simulink model "ctrl_beta_nn"  (R2017a)
settings: Solver=FixedStepAuto  StartTime=0.0  StopTime=20  FixedStep=.001  RelTol=1e-3  EnableMultiTasking=on
settings Model: Creator=aaa  LastModifiedBy=aaa
settings OptimizationCC: LifeSpan=1
settings DebuggingCC: SFExecutionAtInitializationDiag=none

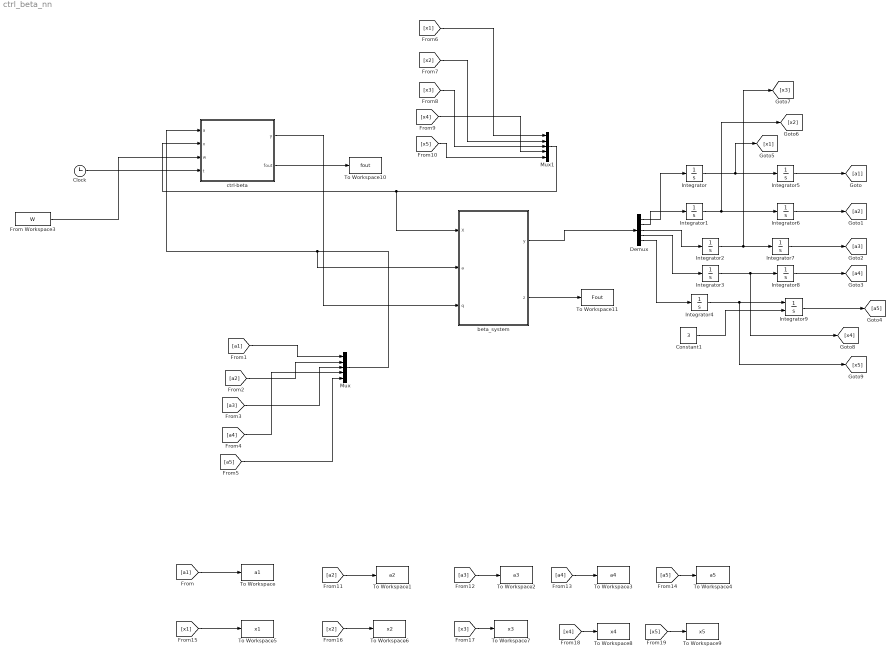
== system ctrl_beta_nn ==
  Clock : Clock
  Constant1 : Constant  Value=3
  Demux : Demux  Outputs=[1 1 1 1 1]
  From Workspace3 : FromWorkspace  VariableName=W  SampleTime=0
  Integrator : Integrator
  Integrator1 : Integrator
  Integrator2 : Integrator  InitialCondition=3.05
  Integrator3 : Integrator  InitialCondition=3
  Integrator4 : Integrator  InitialCondition=1
  Integrator5 : Integrator  InitialCondition=1
  Integrator6 : Integrator  InitialCondition=1
  Integrator7 : Integrator  InitialCondition=pi/6
  Integrator8 : Integrator  InitialCondition=pi/6*5
  Integrator9 : Integrator  InitialConditionSource=external
  Mux : Mux  Inputs=[1 1 1 1 1]
  Mux1 : Mux  Inputs=[1 1 1 1 1]
  To Workspace : ToWorkspace  VariableName=a1  SaveFormat=Timeseries  SampleTime=-1
  To Workspace1 : ToWorkspace  VariableName=a2  SaveFormat=Timeseries  SampleTime=-1
  To Workspace10 : ToWorkspace  VariableName=fout  SaveFormat=Timeseries  SampleTime=-1
  To Workspace11 : ToWorkspace  VariableName=Fout  SaveFormat=Timeseries  SampleTime=-1
  To Workspace2 : ToWorkspace  VariableName=a3  SaveFormat=Timeseries  SampleTime=-1
  To Workspace3 : ToWorkspace  VariableName=a4  SaveFormat=Timeseries  SampleTime=-1
  To Workspace4 : ToWorkspace  VariableName=a5  SaveFormat=Timeseries  SampleTime=-1
  To Workspace5 : ToWorkspace  VariableName=x1  SaveFormat=Timeseries  SampleTime=-1
  To Workspace6 : ToWorkspace  VariableName=x2  SaveFormat=Timeseries  SampleTime=-1
  To Workspace7 : ToWorkspace  VariableName=x3  SaveFormat=Timeseries  SampleTime=-1
  To Workspace8 : ToWorkspace  VariableName=x4  SaveFormat=Timeseries  SampleTime=-1
  To Workspace9 : ToWorkspace  VariableName=x5  SaveFormat=Timeseries  SampleTime=-1
  beta_system : MATLAB Function  TreatAsAtomicUnit=on
  ctrl-beta : MATLAB Function  TreatAsAtomicUnit=on
  wires:
  ctrl-beta/1(y) -> beta_system/3(q)
  Integrator8/1 -> [a4]
  [a3] -> To Workspace2/1
  Integrator6/1 -> [a2]
  From Workspace3/1 -> ctrl-beta/3(w)
  [a4] -> To Workspace3/1
  Integrator9/1 -> [a5]
  [x2] -> Mux1/2
  Integrator3/1 -> [x4], Integrator8/1
  Integrator/1 -> [x1], Integrator5/1
  [x4] -> Mux1/4
  Integrator7/1 -> [a3]
  Mux1/1 -> ctrl-beta/2(x), beta_system/1(X)
  Demux/1 -> Integrator/1
  [a4] -> Mux/4
  [a5] -> Mux/5
  Integrator4/1 -> [x5], Integrator9/1
  Demux/5 -> Integrator4/1
  [a5] -> To Workspace4/1
  [x3] -> To Workspace7/1
  [x4] -> To Workspace8/1
  [a2] -> Mux/2
  [x5] -> To Workspace9/1
  Integrator5/1 -> [a1]
  [a2] -> To Workspace1/1
  [x1] -> Mux1/1
  Demux/4 -> Integrator3/1
  [a3] -> Mux/3
  Demux/3 -> Integrator2/1
  Integrator1/1 -> [x2], Integrator6/1
  [x1] -> To Workspace5/1
  beta_system/1(y) -> Demux/1
  [x3] -> Mux1/3
  Integrator2/1 -> [x3], Integrator7/1
  [a1] -> Mux/1
  Constant1/1 -> Integrator9/2
  [x5] -> Mux1/5
  [a1] -> To Workspace/1
  Mux/1 -> ctrl-beta/1(a), beta_system/2(a)
  Demux/2 -> Integrator1/1
  [x2] -> To Workspace6/1
  ctrl-beta/2(fout) -> To Workspace10/1
  beta_system/2(z) -> To Workspace11/1
  Clock/1 -> ctrl-beta/4(t)

== matlab function ctrl_beta_nn/ctrl-beta ==
  data: a input; x input; y output; w input; fout output; t input
function [y,fout] = fcn(a,x,w,t)

a5=a(5);
x5=x(5);
X=zeros(8,1);
X(1:2)=a(1:2);X(3)=a(5); X(4:8)=x;

num=length(w)-1;
c=X*(1+((1:num)-(num+1)/2)*.05);
sig=sqrt(num+1)/.05;
p=NaN(num,1);
for i=1:num, p(i)=exp(-(X-c(:,i))'*(X-c(:,i))*(sig^2)); end
aaa=0;
fout=w'*[p;1];
y=-10*(x5-aaa)-10*(a5-aaa*t)+fout;

== matlab function ctrl_beta_nn/beta_system ==
  data: X input; y output; a input; q input; z output
function [y,z] = fcn(X,a,q)
% function y = fcn(X,a)
x1=X(1);%dL1
x2=X(2);%dL2
x3=X(3);%dth1
x4=X(4);%dth2
x5=X(5);%dbeta
%NO-Derivative variables as parameters
a1=a(1);a2=a(2);a3=a(3);a4=a(4);a5=a(5);
%other terms
E=1e4; A=1; m=100; w=0.0011; ello=500;
K=E*A/(m*w^2*ello);
th=a3-a4;
L3=(a1^2+a2^2+2*a1*a2*cos(th))^0.5;
e1=1*(a1>1)+0*(a1<=1);
e2=1*(a2>1)+0*(a2<=1);
e3=1*(L3>1)+0*(L3<=1);

%equation
M=[2 cos(th) 0 a2*sin(th) 0;
    cos(th) 2 -a1*sin(th) 0 0;
    0 -a1*sin(th) 2*a1^2 a1*a2*cos(th) 0;
    a2*sin(th) 0 a1*a2*cos(th) 2*a2^2 0;
    0 0 0 0 2*(a1^2*cos(a3)^2+a2^2*cos(a4)^2+a1*a2*cos(a3)*cos(a4))];
N=[2*sin(th)*cos(a5)*x2-2*a1*x3*(x3+2*cos(a5))-a2*cos(a5)*x4*(2*cos(a5)+x4)-(2*a1*cos(a3)+a2*cos(a4))*...
    (2*sin(a5)*sin(a3)+cos(a3)*x5)*x5+2*sin(th)*x2*x4;
    -2*sin(th)*cos(a5)*x1-2*a2*x4*(x4+2*cos(a5))-a1*cos(a5)*x3*(2*cos(a5)+x3)-(2*a2*cos(a4)+a1*cos(a3))*...
    (2*sin(a5)*sin(a4)+cos(a4)*x5)*x5-2*sin(th)*x1*x3;
    4*cos(a5)*a1*x1+2*cos(a5)^2*a1*x2+a1*a2*sin(th)*x4*(2*cos(a5)+x4)+(2*a1*cos(a3)+a2*cos(a4))*...
    (a1*sin(a3)*x5-2*a1*cos(a3)*sin(a5))*x5+4*a1*x1*x3+2*a1*cos(a5)*x2*x4;
    4*cos(a5)*a2*x2+2*cos(a5)^2*a2*x1-a1*a2*sin(th)*x3*(2*cos(a5)+x3)+(2*a2*cos(a4)+a1*cos(a3))*...
    (a2*sin(a4)*x5-2*a2*cos(a4)*sin(a5))*x5+4*a2*x2*x4+2*a2*cos(a5)*x1*x3;
    2*sin(a3)*sin(a5)*(2*a1*cos(a3)+a2*cos(a4))*x1+2*sin(a4)*sin(a5)*(2*a2*cos(a4)+a1*cos(a3))*x2+...
    2*a1*cos(a3)*sin(a5)*(2*a1*cos(a3)+a2*cos(a4))*x3+2*a2*cos(a4)*sin(a5)*(2*a2*cos(a4)+a1*cos(a3))*x4+...
    2*(2*a1*cos(a3)+a2*cos(a4))*cos(a3)*x5*x1+2*(2*a2*cos(a4)+a1*cos(a3))*cos(a4)*x5*x2-...
    2*(2*a1*cos(a3)+a2*cos(a4))*a1*sin(a3)*x3*x5-2*(2*a2*cos(a4)+a1*cos(a3))*a2*sin(a4)*x4*x5];
G=[-cos(a3)*(2*a1*cos(a3)+a2*cos(a4))*(1+2*cos(2*a5));
    -cos(a4)*(2*a2*cos(a4)+a1*cos(a3))*(1+2*cos(2*a5));
    a1*sin(a3)*(2*a1*cos(a3)+a2*cos(a4))*(1+2*cos(2*a5));
    a2*sin(a4)*(2*a2*cos(a4)+a1*cos(a3))*(1+2*cos(2*a5));
    4*(a1^2*cos(a3)^2+a2^2*cos(a4)^2+a1*a2*cos(a3)*cos(a4))*sin(2*a5)];
P=9*K*[(a1-1)*e1+(L3-1)/L3*e3*(a1+a2*cos(th));
    (a2-1)*e2+(L3-1)/L3*e3*(a2+a1*cos(th));
    -(L3-1)*e3*a1*a2/L3*sin(th);
    (L3-1)*e3*a1*a2/L3*sin(th);
    0];

PP=inv(M)*(-N-G-P);

Q=[zeros(4,1); q];
y = PP+Q;
z=-PP(5);
